simulink model "GFLIB_SinCos_BAM_FLT"  (Simulink 8.3)
settings: Solver=ode45  StartTime=0.0  StopTime=10.0  RelTol=1e-3
settings Model: Creator=b37097  LastModifiedBy=B17364
settings DataIOCC: SignalLoggingSaveFormat=Dataset
settings DebuggingCC: UnderspecifiedInitializationDetection=Simplified  StateNameClashWarn=none
settings GRTTargetCC: CombineOutputUpdateFcns=on  GRTInterface=off

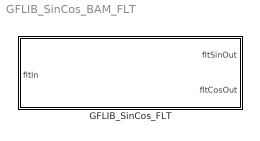
== system GFLIB_SinCos_BAM_FLT ==
  GFLIB_SinCos_FLT : Subsystem  mask(GFLIB_SinCos_FLT){}
      mask help: Bit accurate model of GFLIB_SinCos function, which computes the sin(fltIn) and cos(fltIn) using the floating point optimized approximation.
      mask init:
      | pos = get_param(gcb, 'Position');width = pos(3) - pos(1); height = pos(4) - pos(2);tX=width/2;tY=height*0.9;
      mask Display: color('black');port_label('input',1,'fltIn');port_label('output',1,'fltSinOut');port_label('output',2,'fltCosOut');color('black');disp('GFLIB_SinCos_FLT');color('blue');text(tX,tY, 'BAM', 'horizontalAlignment', 'center');

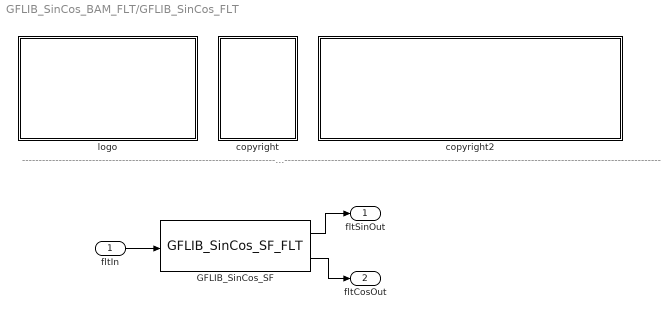
== system GFLIB_SinCos_BAM_FLT/GFLIB_SinCos_FLT ==
  note: ---------------------------------------------------------------------------------------------------------------------------------------------------------------------------------------------------
  fltIn : Inport
  GFLIB_SinCos_SF : S-Function  FunctionName=GFLIB_SinCos_SF_FLT  EnableBusSupport=off
  copyright : Subsystem
      mask Display: text(10,90,'FILE:');text(10,75,'DESRIPTION:');text(10,60,'COPYRIGHT:');text(10,45,'VERSION:');text(10,30,'DATE:')
  copyright2 : Subsystem
      mask Display: text(10,90,'GFLIB_SinCos_BAM_FLT.mdl');text(10,75,'Sine and Cosine transformation');text(10,60,'Freescale');text(10,45,'0.1');text(10,30,'27-Sep-2015');
  logo : Subsystem
      mask Display: image(imread('logo.jpg'))
  fltSinOut : Outport
  fltCosOut : Outport  Port=2
  wires:
  fltIn/1 -> GFLIB_SinCos_SF/1
  GFLIB_SinCos_SF/1 -> fltSinOut/1
  GFLIB_SinCos_SF/2 -> fltCosOut/1

== system GFLIB_SinCos_BAM_FLT/GFLIB_SinCos_FLT/copyright ==

== system GFLIB_SinCos_BAM_FLT/GFLIB_SinCos_FLT/copyright2 ==

== system GFLIB_SinCos_BAM_FLT/GFLIB_SinCos_FLT/logo ==
